simulink model "Wang"  (R2020a)
settings: Solver=VariableStepAuto  StartTime=0.0  StopTime=25  RelTol=1e-3
libraries: simulink x2, Solver_SF x1
settings Model: SimulationMode=accelerator  Creator=wwcong  LastModifiedBy=lennylee
settings DataIOCC: ReturnWorkspaceOutputs=off
settings DebuggingCC: ArithmeticOperatorsInVariantConditions=warning
settings SFSimCC: SimUseLocalCustomCode=off  CustomCodeUndefinedFunction=UseInterfaceOnly
settings RTWCC: RTWUseLocalCustomCode=off

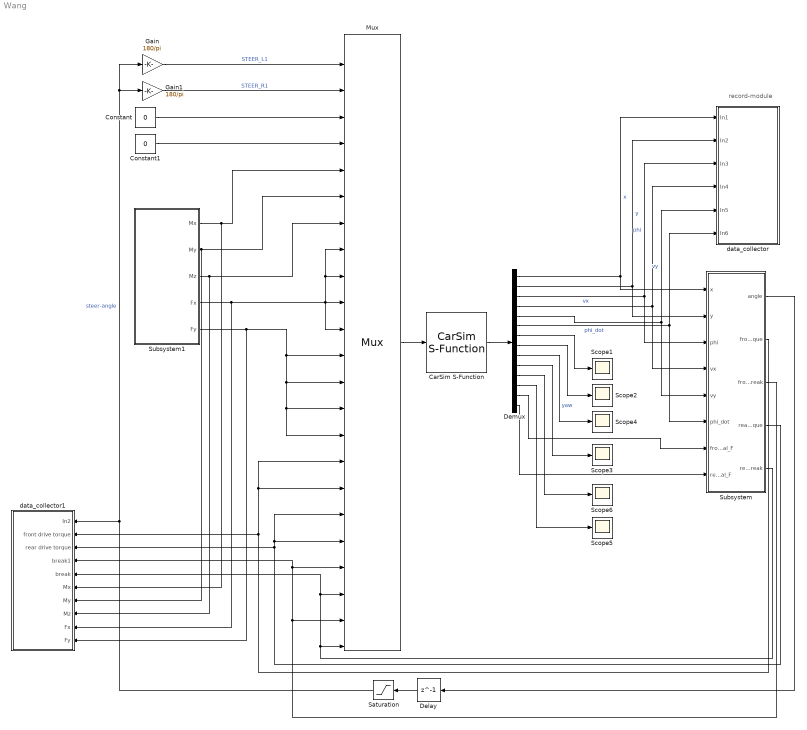
== system Wang ==
  note: record-module
  CarSim S-Function : Solver_SF/CarSim S-Function  Priority=1  SIMFILE=simfile.sim
  Constant : Constant  Value=0
  Constant1 : Constant  Value=0
  Delay : Delay  DelayLength=1  UseCircularBuffer=on
  Demux : Demux  Outputs=14
  Gain : Gain  Gain=180/pi
  Gain1 : Gain  Gain=180/pi
  Mux : Mux  Inputs=24
      settings: DisplayOption=signals
  Saturation : Saturate  UpperLimit=0.7  LowerLimit=-0.7
  Scope{1..6} (6 alike) : Scope
  Subsystem : Subsystem
  Subsystem1 : Subsystem
  data_collector : Subsystem
  data_collector1 : Subsystem
  wires:
  CarSim S-Function/1 -> Demux/1
  Mux/1 -> CarSim S-Function/1
  Demux/1 -> Subsystem/1(x), data_collector/1(In1)  "x"
  Demux/2 -> Subsystem/2(y), data_collector/2(In2)  "y"
  Demux/3 -> Subsystem/3(phi), data_collector/3(In3)  "phi"
  Demux/4 -> Subsystem/4(vx), data_collector/4(In4)  "vx"
  Demux/5 -> Subsystem/5(vy), data_collector/5(In5)  "vy"
  Demux/6 -> Subsystem/6(phi_dot), data_collector/6(In6)  "phi_dot"
  Subsystem/1(angle) -> Delay/1
  Delay/1 -> Saturation/1
  Constant/1 -> Mux/4
  Constant1/1 -> Mux/5
  Saturation/1 -> Gain1/1, Gain/1, data_collector1/1(In2)  "steer-angle"
  Demux/7 -> Scope1/1
  Demux/8 -> Scope2/1
  Demux/9 -> Scope4/1  "yaw"
  Demux/10 -> Scope3/1
  Demux/11 -> Scope6/1
  Demux/12 -> Scope5/1
  Demux/13 -> Subsystem/7(front_vertical_F)
  Demux/14 -> Subsystem/8(rear_vertical_F)
  Subsystem/2(" front drive torque") -> Mux/17, Mux/18, data_collector1/2(" front drive torque")
  Subsystem/3(front break) -> Mux/23, data_collector1/4(break1), Mux/21
  Subsystem/4(rear drive torque) -> Mux/19, Mux/20, data_collector1/3(rear drive torque)
  Subsystem/5(rear break) -> data_collector1/5(break), Mux/22, Mux/24
  Subsystem1/1(Mx) -> data_collector1/6(Mx), Mux/6
  Subsystem1/2(My) -> data_collector1/7(My), Mux/7
  Subsystem1/3(Mz) -> data_collector1/8(Mz), Mux/8
  Subsystem1/4(Fx) -> data_collector1/9(Fx), Mux/9, Mux/10, Mux/12, Mux/11
  Subsystem1/5(Fy) -> data_collector1/10(Fy), Mux/13, Mux/14, Mux/15, Mux/16
  Gain1/1 -> Mux/3  "STEER_R1"
  Gain/1 -> Mux/2  "STEER_L1"

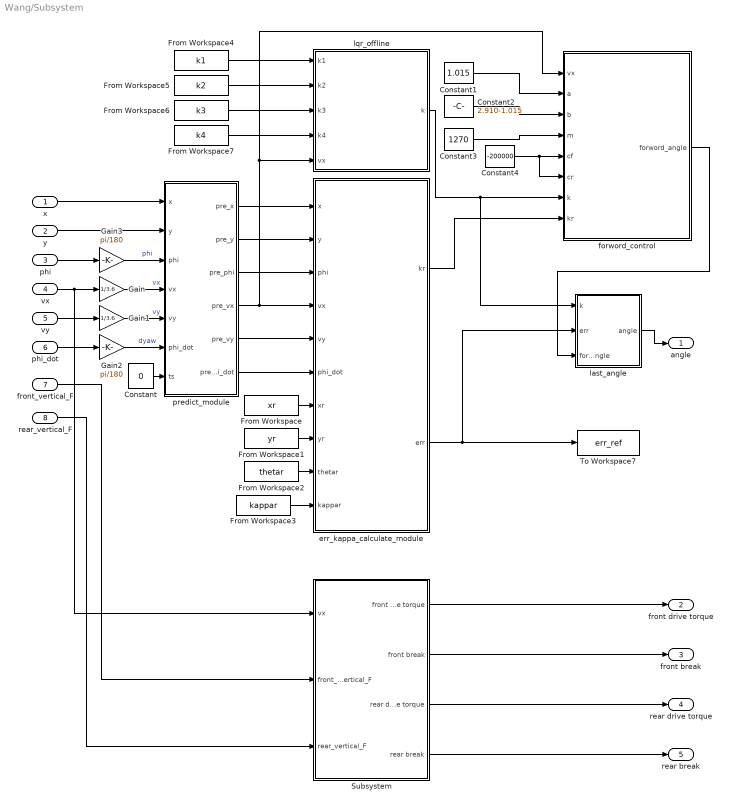
== system Wang/Subsystem ==
  x : Inport
  y : Inport  Port=2
  phi : Inport  Port=3
  vx : Inport  Port=4
  vy : Inport  Port=5
  phi_dot : Inport  Port=6
  front_vertical_F : Inport  Port=7
  rear_vertical_F : Inport  Port=8
  Constant : Constant  Value=0
  Constant1 : Constant  Value=1.015
  Constant2 : Constant  Value=2.910-1.015
  Constant3 : Constant  Value=1270
  Constant4 : Constant  Value=-200000
  From Workspace : FromWorkspace  VariableName=xr
  From Workspace1 : FromWorkspace  VariableName=yr
  From Workspace2 : FromWorkspace  VariableName=thetar
  From Workspace3 : FromWorkspace  VariableName=kappar
  From Workspace4 : FromWorkspace  VariableName=k1
  From Workspace5 : FromWorkspace  VariableName=k2
  From Workspace6 : FromWorkspace  VariableName=k3
  From Workspace7 : FromWorkspace  VariableName=k4
  Gain : Gain  Gain=1/3.6
  Gain1 : Gain  Gain=1/3.6
  Gain2 : Gain  Gain=pi/180
  Gain3 : Gain  Gain=pi/180
  Subsystem : Subsystem
  To Workspace7 : ToWorkspace  VariableName=err_ref  SaveFormat=Timeseries  SampleTime=-1
  err_kappa_calculate_module : MATLAB Function  TreatAsAtomicUnit=on
  forword_control : MATLAB Function  TreatAsAtomicUnit=on
  last_angle : MATLAB Function  TreatAsAtomicUnit=on
  lqr_offline : MATLAB Function  TreatAsAtomicUnit=on
  predict_module : MATLAB Function  TreatAsAtomicUnit=on
  angle : Outport  VectorParamsAs1DForOutWhenUnconnected=off
  " front drive torque" : Outport  Port=2  VectorParamsAs1DForOutWhenUnconnected=off
  front break : Outport  Port=3  VectorParamsAs1DForOutWhenUnconnected=off
  rear drive torque : Outport  Port=4  VectorParamsAs1DForOutWhenUnconnected=off
  rear break : Outport  Port=5  VectorParamsAs1DForOutWhenUnconnected=off
  wires:
  From Workspace7/1 -> lqr_offline/4(k4)
  err_kappa_calculate_module/2(err) -> To Workspace7/1, last_angle/2(err)
  Gain1/1 -> predict_module/5(vy)  "vy"
  From Workspace6/1 -> lqr_offline/3(k3)
  x/1 -> predict_module/1(x)
  lqr_offline/1(k) -> last_angle/1(k), forword_control/7(k)
  phi_dot/1 -> Gain2/1
  predict_module/2(pre_y) -> err_kappa_calculate_module/2(y)
  err_kappa_calculate_module/1(kr) -> forword_control/8(kr)
  forword_control/1(forword_angle) -> last_angle/3(forword_angle)
  predict_module/4(pre_vx) -> lqr_offline/5(vx), forword_control/1(vx), err_kappa_calculate_module/4(vx)
  Gain2/1 -> predict_module/6(phi_dot)  "dyaw"
  last_angle/1(angle) -> angle/1
  phi/1 -> Gain3/1
  From Workspace2/1 -> err_kappa_calculate_module/9(thetar)
  From Workspace5/1 -> lqr_offline/2(k2)
  y/1 -> predict_module/2(y)
  Gain3/1 -> predict_module/3(phi)  "phi"
  From Workspace3/1 -> err_kappa_calculate_module/10(kappar)
  Constant/1 -> predict_module/7(ts)
  From Workspace4/1 -> lqr_offline/1(k1)
  From Workspace1/1 -> err_kappa_calculate_module/8(yr)
  predict_module/1(pre_x) -> err_kappa_calculate_module/1(x)
  predict_module/5(pre_vy) -> err_kappa_calculate_module/5(vy)
  vy/1 -> Gain1/1
  From Workspace/1 -> err_kappa_calculate_module/7(xr)
  predict_module/6(pre_phi_dot) -> err_kappa_calculate_module/6(phi_dot)
  predict_module/3(pre_phi) -> err_kappa_calculate_module/3(phi)
  Constant2/1 -> forword_control/3(b)
  Constant3/1 -> forword_control/4(m)
  Constant4/1 -> forword_control/6(cr), forword_control/5(cf)
  Constant1/1 -> forword_control/2(a)
  Gain/1 -> predict_module/4(vx)  "vx"
  vx/1 -> Subsystem/1(vx), Gain/1
  rear_vertical_F/1 -> Subsystem/3(rear_vertical_F)
  front_vertical_F/1 -> Subsystem/2(front_vertical_F)
  Subsystem/4(rear break) -> rear break/1
  Subsystem/1(" front drive torque") -> " front drive torque"/1
  Subsystem/3(rear drive torque) -> rear drive torque/1
  Subsystem/2(front break) -> front break/1

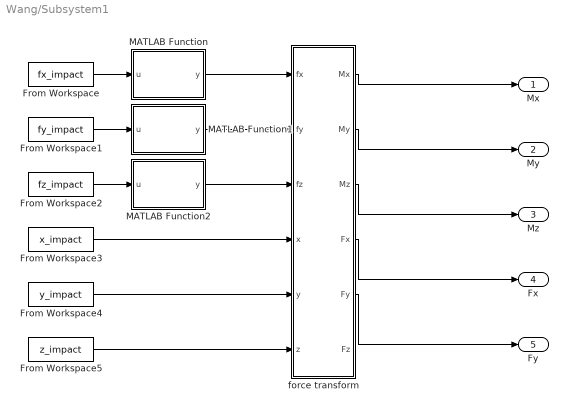
== system Wang/Subsystem1 ==
  From Workspace : FromWorkspace  VariableName=fx_impact
  From Workspace1 : FromWorkspace  VariableName=fy_impact
  From Workspace2 : FromWorkspace  VariableName=fz_impact
  From Workspace3 : FromWorkspace  VariableName=x_impact
  From Workspace4 : FromWorkspace  VariableName=y_impact
  From Workspace5 : FromWorkspace  VariableName=z_impact
  MATLAB Function : MATLAB Function  TreatAsAtomicUnit=on
  MATLAB Function1 : MATLAB Function  TreatAsAtomicUnit=on
  MATLAB Function2 : MATLAB Function  TreatAsAtomicUnit=on
  force transform : MATLAB Function  TreatAsAtomicUnit=on
  Mx : Outport
  My : Outport  Port=2
  Mz : Outport  Port=3
  Fx : Outport  Port=4
  Fy : Outport  Port=5
  wires:
  From Workspace/1 -> MATLAB Function/1(u)
  From Workspace1/1 -> MATLAB Function1/1(u)
  From Workspace2/1 -> MATLAB Function2/1(u)
  MATLAB Function/1(y) -> force transform/1(fx)
  MATLAB Function1/1(y) -> force transform/2(fy)
  MATLAB Function2/1(y) -> force transform/3(fz)
  From Workspace3/1 -> force transform/4(x)
  From Workspace4/1 -> force transform/5(y)
  From Workspace5/1 -> force transform/6(z)
  force transform/5(Fy) -> Fy/1
  force transform/4(Fx) -> Fx/1
  force transform/3(Mz) -> Mz/1
  force transform/2(My) -> My/1
  force transform/1(Mx) -> Mx/1

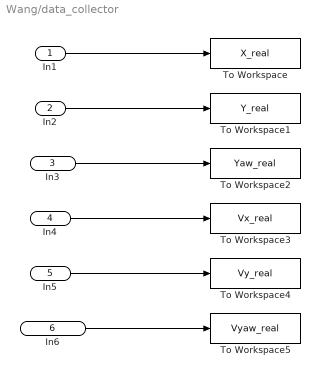
== system Wang/data_collector ==
  In1 : Inport
  In2 : Inport  Port=2
  In3 : Inport  Port=3
  In4 : Inport  Port=4
  In5 : Inport  Port=5
  In6 : Inport  Port=6
  To Workspace : ToWorkspace  VariableName=X_real  SaveFormat=Timeseries  SampleTime=-1
  To Workspace1 : ToWorkspace  VariableName=Y_real  SaveFormat=Timeseries  SampleTime=-1
  To Workspace2 : ToWorkspace  VariableName=Yaw_real  SaveFormat=Timeseries  SampleTime=-1
  To Workspace3 : ToWorkspace  VariableName=Vx_real  SaveFormat=Timeseries  SampleTime=-1
  To Workspace4 : ToWorkspace  VariableName=Vy_real  SaveFormat=Timeseries  SampleTime=-1
  To Workspace5 : ToWorkspace  VariableName=Vyaw_real  SaveFormat=Timeseries  SampleTime=-1
  wires:
  In1/1 -> To Workspace/1
  In2/1 -> To Workspace1/1
  In3/1 -> To Workspace2/1
  In4/1 -> To Workspace3/1
  In5/1 -> To Workspace4/1
  In6/1 -> To Workspace5/1

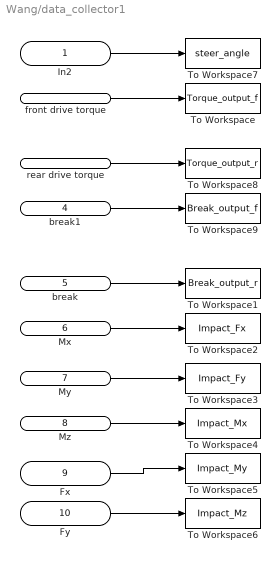
== system Wang/data_collector1 ==
  In2 : Inport
  " front drive torque" : Inport  Port=2
  rear drive torque : Inport  Port=3
  break1 : Inport  Port=4
  break : Inport  Port=5
  Mx : Inport  Port=6
  My : Inport  Port=7
  Mz : Inport  Port=8
  Fx : Inport  Port=9
  Fy : Inport  Port=10
  To Workspace : ToWorkspace  VariableName=Torque_output_f  SaveFormat=Timeseries  SampleTime=-1
  To Workspace1 : ToWorkspace  VariableName=Break_output_r  SaveFormat=Timeseries  SampleTime=-1
  To Workspace2 : ToWorkspace  VariableName=Impact_Fx  SaveFormat=Timeseries  SampleTime=-1
  To Workspace3 : ToWorkspace  VariableName=Impact_Fy  SaveFormat=Timeseries  SampleTime=-1
  To Workspace4 : ToWorkspace  VariableName=Impact_Mx  SaveFormat=Timeseries  SampleTime=-1
  To Workspace5 : ToWorkspace  VariableName=Impact_My  SaveFormat=Timeseries  SampleTime=-1
  To Workspace6 : ToWorkspace  VariableName=Impact_Mz  SaveFormat=Timeseries  SampleTime=-1
  To Workspace7 : ToWorkspace  VariableName=steer_angle  SaveFormat=Timeseries  SampleTime=-1
  To Workspace8 : ToWorkspace  VariableName=Torque_output_r  SaveFormat=Timeseries  SampleTime=-1
  To Workspace9 : ToWorkspace  VariableName=Break_output_f  SaveFormat=Timeseries  SampleTime=-1
  wires:
  My/1 -> To Workspace3/1
  Mx/1 -> To Workspace2/1
  break/1 -> To Workspace1/1
  " front drive torque"/1 -> To Workspace/1
  Fx/1 -> To Workspace5/1
  Mz/1 -> To Workspace4/1
  Fy/1 -> To Workspace6/1
  In2/1 -> To Workspace7/1
  rear drive torque/1 -> To Workspace8/1
  break1/1 -> To Workspace9/1

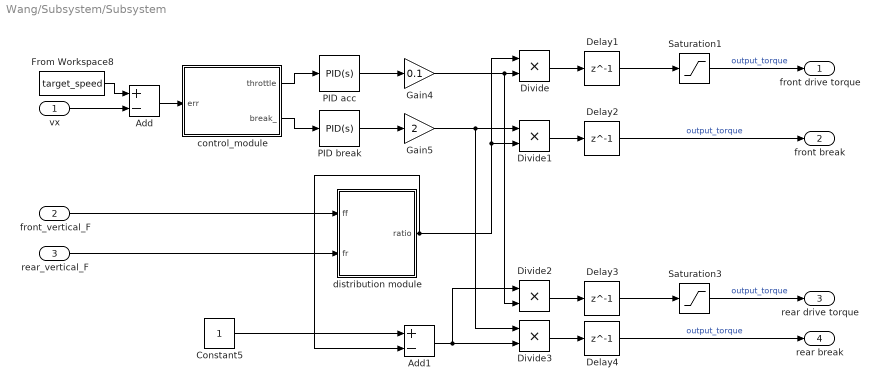
== system Wang/Subsystem/Subsystem ==
  vx : Inport
  front_vertical_F : Inport  Port=2
  rear_vertical_F : Inport  Port=3
  Add : Sum  Inputs=+-
  Add1 : Sum  Inputs=+-
  Constant5 : Constant
  Delay{1..4} (4 alike) : Delay  DelayLength=1  UseCircularBuffer=on
  Divide{,1..3} (4 alike) : Product  Inputs=**
  From Workspace8 : FromWorkspace  VariableName=target_speed
  Gain4 : Gain  Gain=0.1
  Gain5 : Gain  Gain=2
  PID acc : simulink/Continuous/PID Controller  Controller=PID  Form=Parallel  TimeDomain=Continuous-time  UseExternalTs=off  SampleTime=-1  IntegratorMethod=Forward Euler  FilterMethod=Forward Euler  ControllerParametersSource=internal  P=600  I=0  D=0  UseFilter=on  N=0  TunerSelectOption=Transfer Function Based (PID Tuner App)  InitialConditionSource=internal  InitialConditionForIntegrator=0  InitialConditionForFilter=0  DifferentiatorICPrevScaledInput=0  ExternalReset=none  TrackingMode=off  Kt=1  LimitOutput=off  UpperSaturationLimit=inf  LowerSaturationLimit=-inf  LinearizeAsGain=on  AntiWindupMode=none  Kb=1  POutMin=[]  POutMax=[]  IOutMin=[]  IOutMax=[]  DOutMin=[]  DOutMax=[]  NOutMin=[]  NOutMax=[]  SumOutMin=[]  SumOutMax=[]  SaturationOutMin=[]  SaturationOutMax=[]  PParamMin=[]  PParamMax=[]  IParamMin=[]  IParamMax=[]  DParamMin=[]  DParamMax=[]  NParamMin=[]  NParamMax=[]  KbParamMin=[]  KbParamMax=[]  KtParamMin=[]  KtParamMax=[]  KbOutMin=[]  KbOutMax=[]  KtOutMin=[]  KtOutMax=[]  IntegratorOutMin=[]  IntegratorOutMax=[]  FilterOutMin=[]  FilterOutMax=[]  SumI1OutMin=[]  SumI1OutMax=[]  SumI2OutMin=[]  SumI2OutMax=[]  SumI3OutMin=[]  SumI3OutMax=[]  SumI4OutMin=[]  SumI4OutMax=[]  SumDOutMin=[]  SumDOutMax=[]  DifferentiatorOutMin=[]  DifferentiatorOutMax=[]  FilterDiffOutCoefMin=[]  FilterDiffOutCoefMax=[]  ReciprocalOutMin=[]  ReciprocalOutMax=[]  SumDenOutMin=[]  SumDenOutMax=[]  SumNumOutMin=[]  SumNumOutMax=[]  DivideOutMin=[]  DivideOutMax=[]  UdiffTsProdOutMin=[]  UdiffTsProdOutMax=[]  NTsProdOutMin=[]  NTsProdOutMax=[]  UintegralTsProdOutMin=[]  UintegralTsProdOutMax=[]  UngainTsProdOutMin=[]  UngainTsProdOutMax=[]  IntegratorContinuousStateAttributes=''  IntegratorStateMustResolveToSignalObject=off  IntegratorRTWStateStorageClass=Auto  FilterContinuousStateAttributes=''  FilterStateMustResolveToSignalObject=off  FilterRTWStateStorageClass=Auto  ParallelPVariant=InternalParameters  IdealPVariant=Disabled  IVariant=InternalParameters  DVariant=InternalParameters  IntegratorVariant=Continuous  SatVariant=Disabled  AWVariant=Passthrough  PCopyVariant=Disabled  TRVariant=Disabled  FdbkBlocksVariant=Forward  IdealPFdbkVariant=Disabled  SatFdbkVariant=Disabled  DerivativeFilterVariant=ContFilter  NVariant=InternalParameters  NCopyVariant=Disabled  FilterICVariant=InternalICsFilter  IntegratorICVariant=InternalICs  ExternalResetVariant=Disabled  TRSumVariant=Passthrough  SumFdbkVariant=Disabled  SumVariant=Sum_PID  TsampFilterVariant=InternalTs  TsampNgainVariant=Passthrough  TsampIntegralVariant=Passthrough
  PID break : simulink/Continuous/PID Controller  Controller=PID  Form=Parallel  TimeDomain=Continuous-time  UseExternalTs=off  SampleTime=-1  IntegratorMethod=Forward Euler  FilterMethod=Forward Euler  ControllerParametersSource=internal  P=20  I=0  D=1  UseFilter=on  N=0  TunerSelectOption=Transfer Function Based (PID Tuner App)  InitialConditionSource=internal  InitialConditionForIntegrator=0  InitialConditionForFilter=0  DifferentiatorICPrevScaledInput=0  ExternalReset=none  TrackingMode=off  Kt=1  LimitOutput=off  UpperSaturationLimit=inf  LowerSaturationLimit=-inf  LinearizeAsGain=on  AntiWindupMode=none  Kb=1  POutMin=[]  POutMax=[]  IOutMin=[]  IOutMax=[]  DOutMin=[]  DOutMax=[]  NOutMin=[]  NOutMax=[]  SumOutMin=[]  SumOutMax=[]  SaturationOutMin=[]  SaturationOutMax=[]  PParamMin=[]  PParamMax=[]  IParamMin=[]  IParamMax=[]  DParamMin=[]  DParamMax=[]  NParamMin=[]  NParamMax=[]  KbParamMin=[]  KbParamMax=[]  KtParamMin=[]  KtParamMax=[]  KbOutMin=[]  KbOutMax=[]  KtOutMin=[]  KtOutMax=[]  IntegratorOutMin=[]  IntegratorOutMax=[]  FilterOutMin=[]  FilterOutMax=[]  SumI1OutMin=[]  SumI1OutMax=[]  SumI2OutMin=[]  SumI2OutMax=[]  SumI3OutMin=[]  SumI3OutMax=[]  SumI4OutMin=[]  SumI4OutMax=[]  SumDOutMin=[]  SumDOutMax=[]  DifferentiatorOutMin=[]  DifferentiatorOutMax=[]  FilterDiffOutCoefMin=[]  FilterDiffOutCoefMax=[]  ReciprocalOutMin=[]  ReciprocalOutMax=[]  SumDenOutMin=[]  SumDenOutMax=[]  SumNumOutMin=[]  SumNumOutMax=[]  DivideOutMin=[]  DivideOutMax=[]  UdiffTsProdOutMin=[]  UdiffTsProdOutMax=[]  NTsProdOutMin=[]  NTsProdOutMax=[]  UintegralTsProdOutMin=[]  UintegralTsProdOutMax=[]  UngainTsProdOutMin=[]  UngainTsProdOutMax=[]  IntegratorContinuousStateAttributes=''  IntegratorStateMustResolveToSignalObject=off  IntegratorRTWStateStorageClass=Auto  FilterContinuousStateAttributes=''  FilterStateMustResolveToSignalObject=off  FilterRTWStateStorageClass=Auto  ParallelPVariant=InternalParameters  IdealPVariant=Disabled  IVariant=InternalParameters  DVariant=InternalParameters  IntegratorVariant=Continuous  SatVariant=Disabled  AWVariant=Passthrough  PCopyVariant=Disabled  TRVariant=Disabled  FdbkBlocksVariant=Forward  IdealPFdbkVariant=Disabled  SatFdbkVariant=Disabled  DerivativeFilterVariant=ContFilter  NVariant=InternalParameters  NCopyVariant=Disabled  FilterICVariant=InternalICsFilter  IntegratorICVariant=InternalICs  ExternalResetVariant=Disabled  TRSumVariant=Passthrough  SumFdbkVariant=Disabled  SumVariant=Sum_PID  TsampFilterVariant=InternalTs  TsampNgainVariant=Passthrough  TsampIntegralVariant=Passthrough
  Saturation1 : Saturate  UpperLimit=420  LowerLimit=-50
  Saturation3 : Saturate  UpperLimit=420  LowerLimit=-50
  control_module : MATLAB Function  TreatAsAtomicUnit=on
  distribution module : MATLAB Function  TreatAsAtomicUnit=on
  " front drive torque" : Outport  VectorParamsAs1DForOutWhenUnconnected=off
  front break : Outport  Port=2  VectorParamsAs1DForOutWhenUnconnected=off
  rear drive torque : Outport  Port=3  VectorParamsAs1DForOutWhenUnconnected=off
  rear break : Outport  Port=4  VectorParamsAs1DForOutWhenUnconnected=off
  wires:
  Gain5/1 -> Divide3/1, Divide1/1
  Gain4/1 -> Divide2/2, Divide/2
  front_vertical_F/1 -> distribution module/1(ff)
  control_module/2(break_) -> PID break/1
  Add/1 -> control_module/1(err)
  control_module/1(throttle) -> PID acc/1
  From Workspace8/1 -> Add/1
  PID break/1 -> Gain5/1
  PID acc/1 -> Gain4/1
  vx/1 -> Add/2
  distribution module/1(ratio) -> Add1/2, Divide1/2, Divide/1
  rear_vertical_F/1 -> distribution module/2(fr)
  Add1/1 -> Divide2/1, Divide3/2
  Constant5/1 -> Add1/1
  Delay1/1 -> Saturation1/1
  Divide/1 -> Delay1/1
  Saturation1/1 -> " front drive torque"/1  "output_torque"
  Delay2/1 -> front break/1  "output_torque"
  Divide1/1 -> Delay2/1
  Delay3/1 -> Saturation3/1
  Saturation3/1 -> rear drive torque/1  "output_torque"
  Delay4/1 -> rear break/1  "output_torque"
  Divide2/1 -> Delay3/1
  Divide3/1 -> Delay4/1

== matlab function Wang/Subsystem1/MATLAB Function ==
  data: u input; y output
function y = fcn(u)
if(u>0)
    y=u;
else
    y=0;
end

== matlab function Wang/Subsystem1/MATLAB Function1 ==
  data: u input; y output
function y = fcn(u)
if(u>0)
    y=u;
else
    y=0;
end

== matlab function Wang/Subsystem1/MATLAB Function2 ==
  data: u input; y output
function y = fcn(u)
if(u>0)
    y=u;
else
    y=0;
end

== matlab function Wang/Subsystem1/force transform ==
  data: fx input; Mx output; fy input; fz input; x input; y input; z input; My output; Mz output; Fx output; Fy output; Fz output
%%%碰撞力转化方程，需注意这里的力的方向与坐标轴相对应，+与坐标轴方向相同
%%% -则相反
function [Mx,My,Mz,Fx,Fy,Fz] = fcn(fx,fy,fz,x,y,z)
Mz = - fx * y + fy * x;
Mx = - fy * z + fz * y;
My = - fz * x + fx * z;
Fx = fx/4;
Fy = fy/4;
Fz = fz;

== matlab function Wang/Subsystem/err_kappa_calculate_module ==
  data: x input; kr output; y input; phi input; vx input; vy input; phi_dot input; xr input; yr input; thetar input; kappar input; err output
function [kr,err] = fcn(x,y,phi,vx,vy,phi_dot,xr,yr,thetar,kappar)
    n=length(xr);
    d_min=(x-xr(1))^2+(y-yr(1))^2;
    min=1;
    for i=1:n
        d=(x-xr(i))^2+(y-yr(i))^2;
        if d<d_min
            d_min=d;
            min=i;
        end
    end
    dmin=min;
    
    tor=[cos(thetar(dmin));sin(thetar(dmin))];
    nor=[-sin(thetar(dmin));cos(thetar(dmin))];
    d_err=[x-xr(dmin);y-yr(dmin)];
    ed=nor'*d_err;
    es=tor'*d_err;
    %projection_point_thetar=thetar(dmin);%apollo
    projection_point_thetar=thetar(dmin)+kappar(dmin)*es;
    ed_dot=vy*cos(phi-projection_point_thetar)+vx*sin(phi-projection_point_thetar);
    %%%%%%%%%
    ephi=sin(phi-projection_point_thetar);
    %%%%%%%%%
    s_dot=vx*cos(phi-projection_point_thetar)-vy*sin(phi-projection_point_thetar);
    s_dot=s_dot/(1-kappar(dmin)*ed);
    ephi_dot=phi_dot-kappar(dmin)*s_dot;
    kr=kappar(dmin);
    err=[ed;ed_dot;ephi;ephi_dot];
    
    
    
    
    
    
    
    
    
    
    
    


end

== matlab function Wang/Subsystem/predict_module ==
  data: x input; pre_x output; y input; phi input; vx input; vy input; phi_dot input; ts input; pre_y output; pre_phi output; pre_vx output; pre_vy output; pre_phi_dot output
function [pre_x,pre_y,pre_phi,pre_vx,pre_vy,pre_phi_dot] = fcn(x,y,phi,vx,vy,phi_dot,ts)
    pre_x=x+vx*ts*cos(phi)-vy*ts*sin(phi);
    pre_y=y+vy*ts*cos(phi)+vx*ts*sin(phi);
    pre_phi=phi+phi_dot*ts;
    pre_vx=vx;
    pre_vy=vy;
    pre_phi_dot=phi_dot;
end

== matlab function Wang/Subsystem/lqr_offline ==
  data: k1 input; k output; k2 input; k3 input; k4 input; vx input
function k  = fcn(k1,k2,k3,k4,vx)
    if vx<0.01
        k=[0,0,0,0];
    else
        index=round(vx/0.01);
        k=[k1(index),k2(index),k3(index),k4(index)];
    end
end

== matlab function Wang/Subsystem/forword_control ==
  data: vx input; a input; forword_angle output; b input; m input; cf input; cr input; k input; kr input
function forword_angle = fcn(vx,a,b,m,cf,cr,k,kr)
    forword_angle=kr*(a+b-b*k(3)-(m*vx*vx/(a+b))*((b/cf)+(a/cr)*k(3)-(a/cr)));
end

== matlab function Wang/Subsystem/last_angle ==
  data: k input; angle output; err input; forword_angle input
function angle = fcn(k,err,forword_angle)

    angle=-k*err+forword_angle;
end

== matlab function Wang/Subsystem/Subsystem/control_module ==
  data: err input; throttle output; break_ output
function [throttle, break_] = fcn(err)
%%%
%accelerate or brak
%%%
if(err>=0)
    throttle = err;
    break_ = 0;
else
    break_ = -err;
    throttle =0;
end

== matlab function Wang/Subsystem/Subsystem/distribution module ==
  data: ff input; ratio output; fr input
function ratio = fcn(ff,fr)

    ratio=ff/(ff+fr);
end
